simulink model "exsim3modelPart2d"  (R2018b)
settings: Solver=VariableStepAuto  StartTime=0.0  StopTime=10.0  RelTol=1e-3
values from neighbouring files (symbols this model uses):
  gamma = 0.01    [exsim3.m]
  Kcss = 3    [exsim3.m]
  nb = eval(solutionKb(2))    [exsim3.m]
  Ts = 0.2    [exsim3.m]
libraries: simulink x1
settings Model: Creator=rafael  LastModifiedBy=rafael

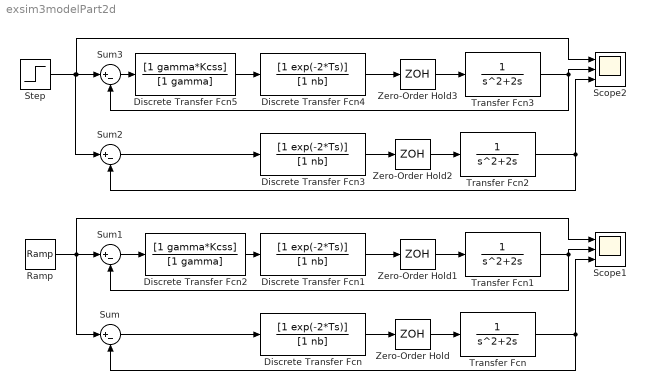
== system exsim3modelPart2d ==
  Discrete Transfer Fcn{,1,3..4} (4 alike) : DiscreteTransferFcn  Numerator=[1 exp(-2*Ts)]  Denominator=[1 nb]  SampleTime=Ts
  Discrete Transfer Fcn2 : DiscreteTransferFcn  Numerator=[1 gamma*Kcss]  Denominator=[1 gamma]  SampleTime=Ts
  Discrete Transfer Fcn5 : DiscreteTransferFcn  Numerator=[1 gamma*Kcss]  Denominator=[1 gamma]  SampleTime=Ts
  Ramp : simulink/Sources/Ramp  slope=1  start=0  InitialOutput=0
  Scope1 : Scope  NumInputPorts=3
  Scope2 : Scope  NumInputPorts=3
  Step : Step  SampleTime=0
  Sum{,1..3} (4 alike) : Sum  Inputs=|+-
  Transfer Fcn{,1..3} (4 alike) : TransferFcn  Denominator=[1 2 0]
  Zero-Order Hold{,1..3} (4 alike) : ZeroOrderHold  SampleTime=Ts
  wires:
  Zero-Order Hold/1 -> Transfer Fcn/1
  Discrete Transfer Fcn/1 -> Zero-Order Hold/1
  Sum/1 -> Discrete Transfer Fcn/1
  Transfer Fcn/1 -> Scope1/3, Sum/2
  Ramp/1 -> Sum/1, Sum1/1, Scope1/1
  Discrete Transfer Fcn1/1 -> Zero-Order Hold1/1
  Transfer Fcn1/1 -> Sum1/2, Scope1/2
  Zero-Order Hold1/1 -> Transfer Fcn1/1
  Sum1/1 -> Discrete Transfer Fcn2/1
  Discrete Transfer Fcn2/1 -> Discrete Transfer Fcn1/1
  Transfer Fcn2/1 -> Scope2/3, Sum2/2
  Discrete Transfer Fcn3/1 -> Zero-Order Hold2/1
  Zero-Order Hold2/1 -> Transfer Fcn2/1
  Step/1 -> Sum2/1, Scope2/1, Sum3/1
  Discrete Transfer Fcn4/1 -> Zero-Order Hold3/1
  Transfer Fcn3/1 -> Sum3/2, Scope2/2
  Sum2/1 -> Discrete Transfer Fcn3/1
  Zero-Order Hold3/1 -> Transfer Fcn3/1
  Sum3/1 -> Discrete Transfer Fcn5/1
  Discrete Transfer Fcn5/1 -> Discrete Transfer Fcn4/1
